simulink model "chapter2_4"  (R2022a)
settings: Solver=FixedStepAuto  StartTime=0.0  StopTime=8  FixedStep=1e-3  RelTol=1e-3
model workspace (MAT data in the model file):
  maxRandom = 1e-06
  minRandom = -1e-06
values from neighbouring files (symbols this model uses):
  A = A_set(N1-5)    [Figure2_12and2_13.m]    (also in Figure2_3.m = 10; Figure2_9and2_10and2_11.m; parameterLoadForchapter2_4.m = 0.0005; parameterLoadForchapter2_5.m = 0.0005)
  Cb = 11e3    (= 11000)    [parameterLoadForchapter2_4.m]    (also in parameterLoadForchapter2_5.m)
  Cv = 5000    [parameterLoadForchapter2_4.m]    (also in parameterLoadForchapter2_5.m)
  d = 2.6    [parameterLoadForchapter2_4.m]    (also in parameterLoadForchapter2_5.m; parameter_load3.m)
  Jb = 927.8    [parameterLoadForchapter2_4.m]    (also in parameterLoadForchapter2_5.m)
  Jv = 3044    [parameterLoadForchapter2_4.m]    (also in parameterLoadForchapter2_5.m)
  Kb = 0.267e6    (= 267000)    [parameterLoadForchapter2_4.m]    (also in parameterLoadForchapter2_5.m)
  Kv = 1.5e6    (= 1500000)    [parameterLoadForchapter2_4.m]    (also in parameterLoadForchapter2_5.m)
  L = 210/2    (= 105)    [Figure2_18_and2_19.m]    (also in Figure2_20_and2_21.m; parameterLoadForchapter2_4.m = 15.6; parameterLoadForchapter2_5.m = 210; parameter_load3.m = 210)
  Mb = 23000    [parameterLoadForchapter2_4.m]    (also in parameterLoadForchapter2_5.m)
  Mv = 4060    [parameterLoadForchapter2_4.m]    (also in parameterLoadForchapter2_5.m)
  mw = 1670    [parameterLoadForchapter2_4.m]    (also in parameterLoadForchapter2_5.m)
  Mw = 1670    [parameterLoadForchapter2_4.m]    (also in parameterLoadForchapter2_5.m)
  N1 = 0    [Mchapter2_5.m]
  N2 = N    [Figure2_10and2_11.m]    (also in Figure2_12and2_13.m = N1; Figure2_7and2_8and2_9.m = 0; Figure2_9and2_10and2_11.m = 0; Mchapter2_5.m = 0)
  r = 0.42    [parameterLoadForchapter2_4.m]    (also in parameterLoadForchapter2_5.m; parameter_load3.m)
  v = 100/3.6    (= 27.7777777778)    [Figure2_18_and2_19.m]    (also in Figure2_20_and2_21.m; parameterLoadForchapter2_4.m = 13.8888888889; parameterLoadForchapter2_5.m; parameter_load3.m)
settings Model: Creator=Spicydel  LastModifiedBy=Spicydel

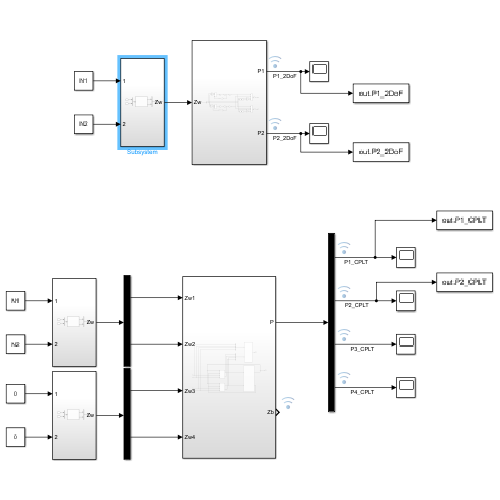
[thumbnail: Simulink's stored preview of the top-level diagram]
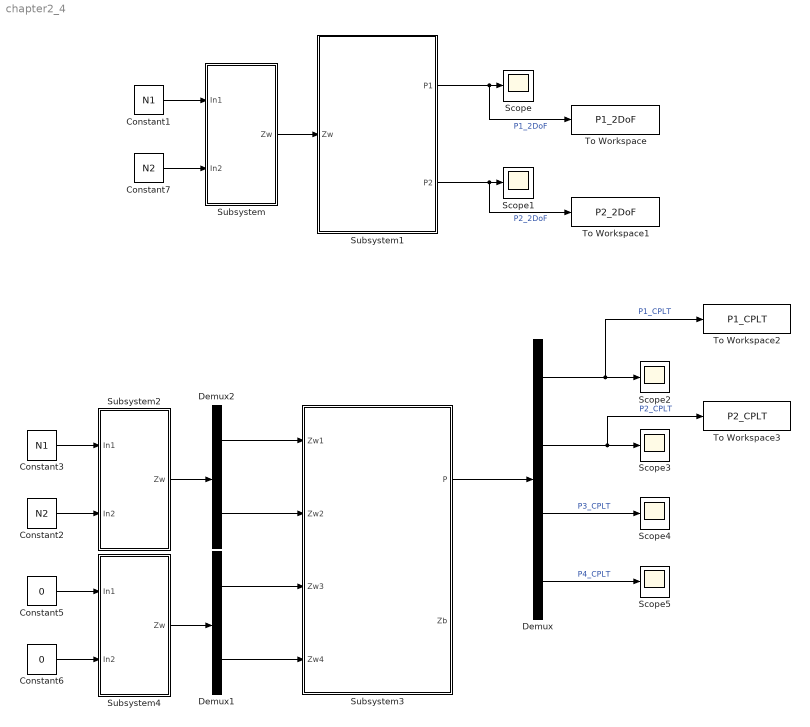
== system chapter2_4 ==
  Constant1 : Constant  Value=N1
  Constant2 : Constant  Value=N2
  Constant3 : Constant  Value=N1
  Constant5 : Constant  Value=0
  Constant6 : Constant  Value=0
  Constant7 : Constant  Value=N2
  Demux : Demux
  Demux1 : Demux  Outputs=2
  Demux2 : Demux  Outputs=2
  Scope{,1..5} (6 alike) : Scope
  Subsystem : Subsystem
  Subsystem1 : Subsystem
  Subsystem2 : Subsystem
  Subsystem3 : Subsystem
  Subsystem4 : Subsystem
  To Workspace : ToWorkspace  VariableName=P1_2DoF  SaveFormat=Timeseries  SampleTime=-1
  To Workspace1 : ToWorkspace  VariableName=P2_2DoF  SaveFormat=Timeseries  SampleTime=-1
  To Workspace2 : ToWorkspace  VariableName=P1_CPLT  SaveFormat=Timeseries  SampleTime=-1
  To Workspace3 : ToWorkspace  VariableName=P2_CPLT  SaveFormat=Timeseries  SampleTime=-1
  wires:
  Constant1/1 -> Subsystem/1(In1)
  Constant7/1 -> Subsystem/2(In2)
  Subsystem/1(Zw) -> Subsystem1/1(Zw)
  Subsystem1/1(P1) -> To Workspace/1, Scope/1  "P1_2DoF"
  Subsystem1/2(P2) -> To Workspace1/1, Scope1/1  "P2_2DoF"
  Subsystem2/1(Zw) -> Demux2/1
  Constant2/1 -> Subsystem2/2(In2)
  Constant3/1 -> Subsystem2/1(In1)
  Constant5/1 -> Subsystem4/1(In1)
  Constant6/1 -> Subsystem4/2(In2)
  Subsystem4/1(Zw) -> Demux1/1
  Demux1/1 -> Subsystem3/3(Zw3)
  Demux1/2 -> Subsystem3/4(Zw4)
  Demux2/1 -> Subsystem3/1(Zw1)
  Demux2/2 -> Subsystem3/2(Zw2)
  Subsystem3/1(P) -> Demux/1
  Demux/1 -> To Workspace2/1, Scope2/1  "P1_CPLT"
  Demux/2 -> To Workspace3/1, Scope3/1  "P2_CPLT"
  Demux/3 -> Scope4/1  "P3_CPLT"
  Demux/4 -> Scope5/1  "P4_CPLT"

== system chapter2_4/Subsystem ==
  In1 : Inport
  In2 : Inport  Port=2
  Mux1 : Mux  Inputs=2
  Mux2 : Mux  Inputs=2
  poly : Subsystem
  Zw : Outport
  wires:
  poly/1(wheel1) -> Mux2/1
  In2/1 -> Mux1/2
  poly/2(wheel2) -> Mux2/2
  Mux1/1 -> poly/1(N)
  In1/1 -> Mux1/1
  Mux2/1 -> Zw/1

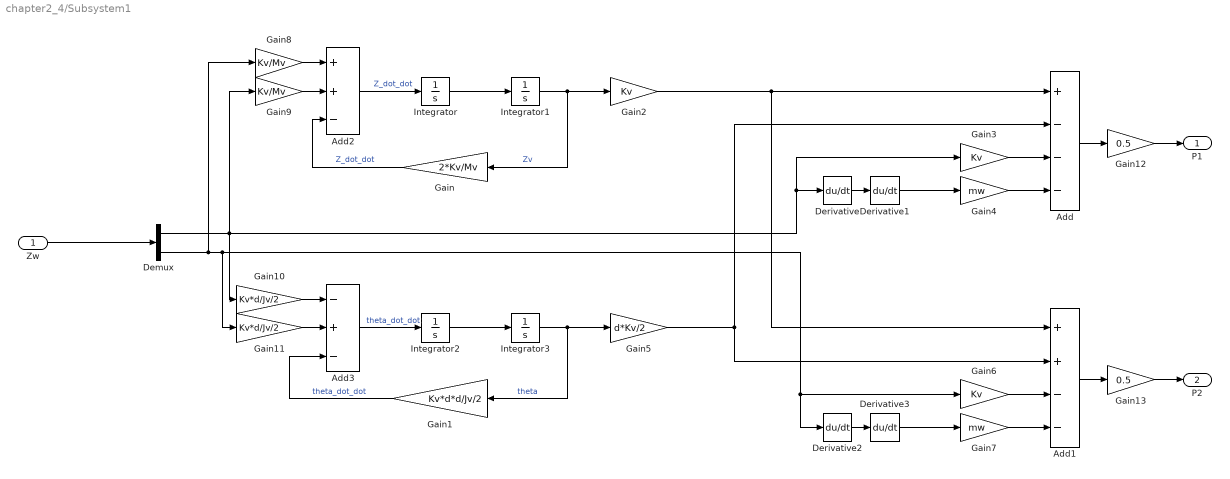
== system chapter2_4/Subsystem1 ==
  Zw : Inport
  Add : Sum  Inputs=+---
  Add1 : Sum  Inputs=++--
  Add2 : Sum  Inputs=++-
  Add3 : Sum  Inputs=-+-
  Demux : Demux  Outputs=2
  Derivative{,1..3} (4 alike) : Derivative
  Gain : Gain  Gain=2*Kv/Mv
  Gain1 : Gain  Gain=Kv*d*d/Jv/2
  Gain10 : Gain  Gain=Kv*d/Jv/2
  Gain11 : Gain  Gain=Kv*d/Jv/2
  Gain12 : Gain  Gain=0.5
  Gain13 : Gain  Gain=0.5
  Gain2 : Gain  Gain=Kv
  Gain3 : Gain  Gain=Kv
  Gain4 : Gain  Gain=mw
  Gain5 : Gain  Gain=d*Kv/2
  Gain6 : Gain  Gain=Kv
  Gain7 : Gain  Gain=mw
  Gain8 : Gain  Gain=Kv/Mv
  Gain9 : Gain  Gain=Kv/Mv
  Integrator{,1..3} (4 alike) : Integrator
  P1 : Outport
  P2 : Outport  Port=2
  wires:
  Integrator/1 -> Integrator1/1
  Integrator1/1 -> Gain2/1, Gain/1  "Zv"
  Add2/1 -> Integrator/1  "Z_dot_dot"
  Integrator2/1 -> Integrator3/1
  Integrator3/1 -> Gain5/1, Gain1/1  "theta"
  Add3/1 -> Integrator2/1  "theta_dot_dot"
  Gain2/1 -> Add1/1, Add/1
  Gain5/1 -> Add/2, Add1/2
  Add/1 -> Gain12/1
  Add1/1 -> Gain13/1
  Zw/1 -> Demux/1
  Demux/1 -> Gain10/1, Gain9/1, Derivative/1, Gain3/1
  Gain3/1 -> Add/3
  Derivative/1 -> Derivative1/1
  Derivative1/1 -> Gain4/1
  Gain4/1 -> Add/4
  Demux/2 -> Gain11/1, Gain6/1, Derivative2/1, Gain8/1
  Gain6/1 -> Add1/3
  Derivative2/1 -> Derivative3/1
  Derivative3/1 -> Gain7/1
  Gain7/1 -> Add1/4
  Gain/1 -> Add2/3  "Z_dot_dot"
  Gain8/1 -> Add2/1
  Gain9/1 -> Add2/2
  Gain1/1 -> Add3/3  "theta_dot_dot"
  Gain10/1 -> Add3/1
  Gain11/1 -> Add3/2
  Gain12/1 -> P1/1
  Gain13/1 -> P2/1

== system chapter2_4/Subsystem2 ==
  In1 : Inport
  In2 : Inport  Port=2
  Mux1 : Mux  Inputs=2
  Mux2 : Mux  Inputs=2
  poly : Subsystem
  Zw : Outport
  wires:
  Mux2/1 -> Zw/1
  In1/1 -> Mux1/1
  Mux1/1 -> poly/1(N)
  poly/2(wheel2) -> Mux2/2
  In2/1 -> Mux1/2
  poly/1(wheel1) -> Mux2/1

== system chapter2_4/Subsystem3 ==
  Zw1 : Inport
  Zw2 : Inport  Port=2
  Zw3 : Inport  Port=3
  Zw4 : Inport  Port=4
  FrontTrans : Subsystem
  Mux : Mux
  Mux1 : Mux
  RearTrans : Subsystem
  Subsystem : Subsystem
  Subsystem2 : Subsystem
  P : Outport
  Zb : Outport  Port=2
  wires:
  RearTrans/1(Zv2) -> Mux1/3, Subsystem2/2(Zv2)
  FrontTrans/1(Zv1) -> Mux1/1, Subsystem2/1(Zv1)
  Subsystem2/1(Zb) -> Zb/1, RearTrans/1(Zb), FrontTrans/1(Zb)  "Zb"
  Zw4/1 -> Mux/4, RearTrans/4(Zw4)
  Subsystem2/2(theta_b) -> FrontTrans/2(theta_b), RearTrans/2(theta_b)
  Zw3/1 -> Mux/3, RearTrans/3(Zw3)
  Zw1/1 -> Mux/1, FrontTrans/3(Zw1)
  Zw2/1 -> Mux/2, FrontTrans/4(Zw2)
  FrontTrans/2(theta_v1) -> Mux1/2
  RearTrans/2(theta_v2) -> Mux1/4
  Mux/1 -> Subsystem/1(Zw)
  Mux1/1 -> Subsystem/2(Z&theta)
  Subsystem/1(P) -> P/1

== system chapter2_4/Subsystem4 ==
  In1 : Inport
  In2 : Inport  Port=2
  Mux1 : Mux  Inputs=2
  Mux2 : Mux  Inputs=2
  poly : Subsystem
  Zw : Outport
  wires:
  poly/1(wheel1) -> Mux2/1
  In2/1 -> Mux1/2
  poly/2(wheel2) -> Mux2/2
  Mux1/1 -> poly/1(N)
  In1/1 -> Mux1/1
  Mux2/1 -> Zw/1

== system chapter2_4/Subsystem/poly ==
  N : Inport
  Clock : Clock
  Constant : Constant  Value=v
  Demux : Demux  Outputs=2
  Gain1 : Gain  Gain=1/r
  Product1 : Product
  Subsystem : Subsystem
  Subsystem1 : Subsystem
  wheel1 : Outport
  wheel2 : Outport  Port=2
  wires:
  Constant/1 -> Gain1/1
  Gain1/1 -> Product1/1
  Clock/1 -> Product1/2
  Product1/1 -> [omega]
  [omega] -> Subsystem/2(In2)
  Subsystem/1(Out1) -> wheel1/1
  [omega] -> Subsystem1/2(In2)
  Subsystem1/1(Out1) -> wheel2/1
  N/1 -> Demux/1
  Demux/1 -> Subsystem/1(In1)
  Demux/2 -> Subsystem1/1(In1)

== system chapter2_4/Subsystem2/poly ==
  N : Inport
  Clock : Clock
  Constant : Constant  Value=v
  Demux : Demux  Outputs=2
  Gain1 : Gain  Gain=1/r
  Product1 : Product
  Subsystem : Subsystem
  Subsystem1 : Subsystem
  wheel1 : Outport
  wheel2 : Outport  Port=2
  wires:
  Demux/2 -> Subsystem1/1(In1)
  Demux/1 -> Subsystem/1(In1)
  N/1 -> Demux/1
  Subsystem1/1(Out1) -> wheel2/1
  [omega] -> Subsystem1/2(In2)
  Subsystem/1(Out1) -> wheel1/1
  [omega] -> Subsystem/2(In2)
  Product1/1 -> [omega]
  Clock/1 -> Product1/2
  Gain1/1 -> Product1/1
  Constant/1 -> Gain1/1

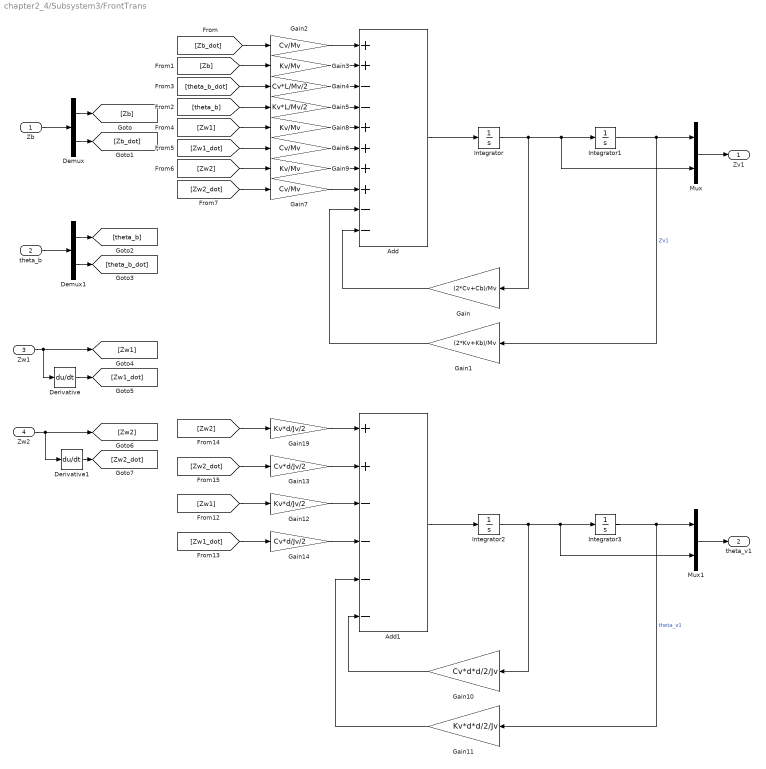
== system chapter2_4/Subsystem3/FrontTrans ==
  Zb : Inport
  theta_b : Inport  Port=2
  Zw1 : Inport  Port=3
  Zw2 : Inport  Port=4
  Add : Sum  Inputs=++--++++--
  Add1 : Sum  Inputs=++----
  Demux : Demux  Outputs=2
  Demux1 : Demux  Outputs=2
  Derivative : Derivative
  Derivative1 : Derivative
  Gain : Gain  Gain=(2*Cv+Cb)/Mv
  Gain1 : Gain  Gain=(2*Kv+Kb)/Mv
  Gain10 : Gain  Gain=Cv*d*d/2/Jv
  Gain11 : Gain  Gain=Kv*d*d/2/Jv
  Gain12 : Gain  Gain=Kv*d/Jv/2
  Gain13 : Gain  Gain=Cv*d/Jv/2
  Gain14 : Gain  Gain=Cv*d/Jv/2
  Gain19 : Gain  Gain=Kv*d/Jv/2
  Gain2 : Gain  Gain=Cv/Mv
  Gain3 : Gain  Gain=Kv/Mv
  Gain4 : Gain  Gain=Cv*L/Mv/2
  Gain5 : Gain  Gain=Kv*L/Mv/2
  Gain6 : Gain  Gain=Cv/Mv
  Gain7 : Gain  Gain=Cv/Mv
  Gain8 : Gain  Gain=Kv/Mv
  Gain9 : Gain  Gain=Kv/Mv
  Integrator{,1..3} (4 alike) : Integrator
  Mux : Mux  Inputs=2
  Mux1 : Mux  Inputs=2
  Zv1 : Outport
  theta_v1 : Outport  Port=2
  wires:
  Zb/1 -> Demux/1
  theta_b/1 -> Demux1/1
  Demux/1 -> [Zb]
  Demux/2 -> [Zb_dot]
  Demux1/1 -> [theta_b]
  Demux1/2 -> [theta_b_dot]
  Integrator/1 -> Gain/1, Mux/2, Integrator1/1
  Add/1 -> Integrator/1
  Integrator1/1 -> Gain1/1, Mux/1  "Zv1"
  Mux/1 -> Zv1/1
  Zw1/1 -> [Zw1], Derivative/1
  Gain/1 -> Add/10
  Gain1/1 -> Add/9
  [Zb_dot] -> Gain2/1
  Gain2/1 -> Add/1
  [Zb] -> Gain3/1
  Gain3/1 -> Add/2
  [theta_b_dot] -> Gain4/1
  Gain4/1 -> Add/3
  [theta_b] -> Gain5/1
  Gain5/1 -> Add/4
  [Zw2] -> Gain9/1
  [Zw2_dot] -> Gain7/1
  [Zw1_dot] -> Gain6/1
  [Zw1] -> Gain8/1
  Gain8/1 -> Add/5
  Gain6/1 -> Add/6
  Gain9/1 -> Add/7
  Gain7/1 -> Add/8
  [Zw1] -> Gain12/1
  [Zw1_dot] -> Gain14/1
  [Zw2_dot] -> Gain13/1
  [Zw2] -> Gain19/1
  Gain11/1 -> Add1/5
  Gain10/1 -> Add1/6
  Add1/1 -> Integrator2/1
  Gain19/1 -> Add1/1
  Gain12/1 -> Add1/3
  Gain13/1 -> Add1/2
  Gain14/1 -> Add1/4
  Mux1/1 -> theta_v1/1
  Integrator3/1 -> Mux1/1, Gain11/1  "theta_v1"
  Integrator2/1 -> Mux1/2, Integrator3/1, Gain10/1
  Derivative/1 -> [Zw1_dot]
  Zw2/1 -> [Zw2], Derivative1/1
  Derivative1/1 -> [Zw2_dot]

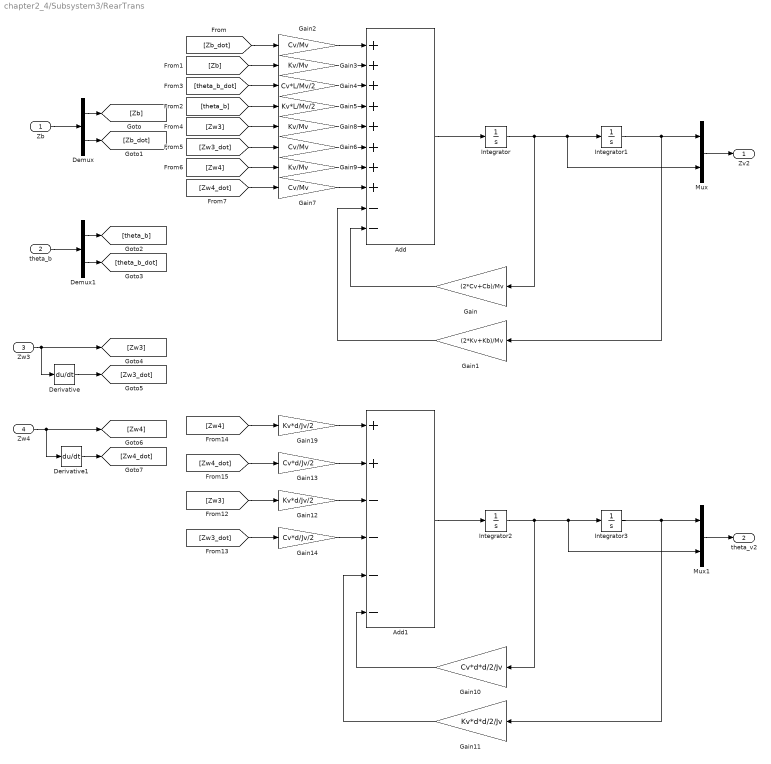
== system chapter2_4/Subsystem3/RearTrans ==
  Zb : Inport
  theta_b : Inport  Port=2
  Zw3 : Inport  Port=3
  Zw4 : Inport  Port=4
  Add : Sum  Inputs=++++++++--
  Add1 : Sum  Inputs=++----
  Demux : Demux  Outputs=2
  Demux1 : Demux  Outputs=2
  Derivative : Derivative
  Derivative1 : Derivative
  Gain : Gain  Gain=(2*Cv+Cb)/Mv
  Gain1 : Gain  Gain=(2*Kv+Kb)/Mv
  Gain10 : Gain  Gain=Cv*d*d/2/Jv
  Gain11 : Gain  Gain=Kv*d*d/2/Jv
  Gain12 : Gain  Gain=Kv*d/Jv/2
  Gain13 : Gain  Gain=Cv*d/Jv/2
  Gain14 : Gain  Gain=Cv*d/Jv/2
  Gain19 : Gain  Gain=Kv*d/Jv/2
  Gain2 : Gain  Gain=Cv/Mv
  Gain3 : Gain  Gain=Kv/Mv
  Gain4 : Gain  Gain=Cv*L/Mv/2
  Gain5 : Gain  Gain=Kv*L/Mv/2
  Gain6 : Gain  Gain=Cv/Mv
  Gain7 : Gain  Gain=Cv/Mv
  Gain8 : Gain  Gain=Kv/Mv
  Gain9 : Gain  Gain=Kv/Mv
  Integrator{,1..3} (4 alike) : Integrator
  Mux : Mux  Inputs=2
  Mux1 : Mux  Inputs=2
  Zv2 : Outport
  theta_v2 : Outport  Port=2
  wires:
  Gain14/1 -> Add1/4
  Gain13/1 -> Add1/2
  Gain12/1 -> Add1/3
  Gain19/1 -> Add1/1
  Add1/1 -> Integrator2/1
  Gain10/1 -> Add1/6
  Gain11/1 -> Add1/5
  [Zw4] -> Gain19/1
  [Zw4_dot] -> Gain13/1
  [Zw3_dot] -> Gain14/1
  [Zw3] -> Gain12/1
  Gain7/1 -> Add/8
  Gain9/1 -> Add/7
  Gain6/1 -> Add/6
  Gain8/1 -> Add/5
  [Zw3] -> Gain8/1
  [Zw3_dot] -> Gain6/1
  [Zw4_dot] -> Gain7/1
  [Zw4] -> Gain9/1
  Gain5/1 -> Add/4
  [theta_b] -> Gain5/1
  Gain4/1 -> Add/3
  [theta_b_dot] -> Gain4/1
  Gain3/1 -> Add/2
  [Zb] -> Gain3/1
  Gain2/1 -> Add/1
  [Zb_dot] -> Gain2/1
  Gain1/1 -> Add/9
  Gain/1 -> Add/10
  Zw4/1 -> Derivative1/1, [Zw4]
  Derivative1/1 -> [Zw4_dot]
  Zw3/1 -> Derivative/1, [Zw3]
  Mux/1 -> Zv2/1
  Integrator1/1 -> Mux/1, Gain1/1
  Add/1 -> Integrator/1
  Integrator/1 -> Integrator1/1, Mux/2, Gain/1
  Demux1/2 -> [theta_b_dot]
  Demux1/1 -> [theta_b]
  Demux/2 -> [Zb_dot]
  Demux/1 -> [Zb]
  theta_b/1 -> Demux1/1
  Zb/1 -> Demux/1
  Integrator2/1 -> Gain10/1, Mux1/2, Integrator3/1
  Integrator3/1 -> Mux1/1, Gain11/1
  Mux1/1 -> theta_v2/1
  Derivative/1 -> [Zw3_dot]

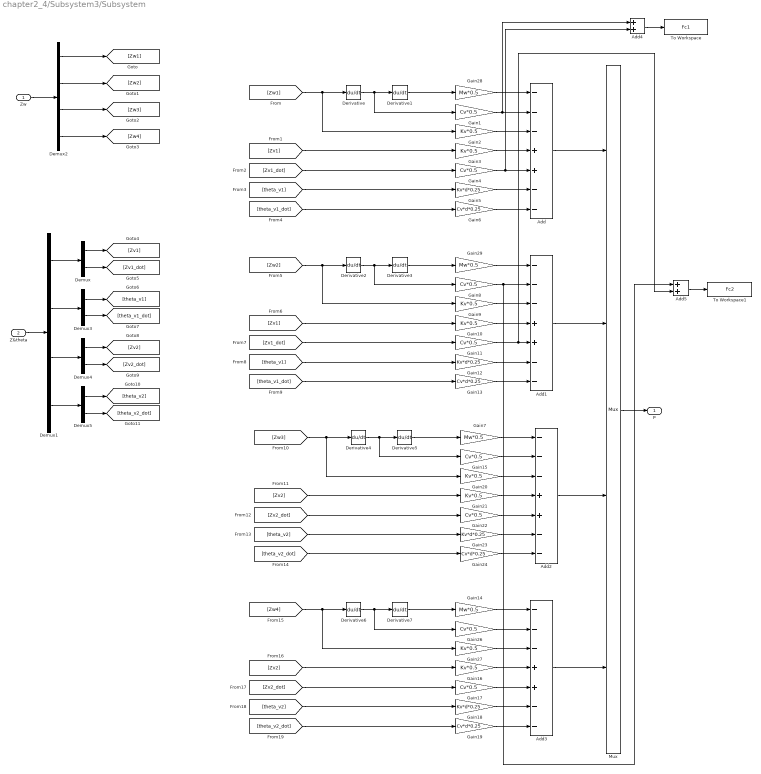
== system chapter2_4/Subsystem3/Subsystem ==
  Zw : Inport
  Z&theta : Inport  Port=2
  Add{,1..3} (4 alike) : Sum  Inputs=---++--
  Add4 : Sum
  Add5 : Sum
  Demux{,3..5} (4 alike) : Demux  Outputs=2
  Demux1 : Demux
  Demux2 : Demux
  Derivative{,1..7} (8 alike) : Derivative
  Gain{1,4,8,11,15,17,22,26} (8 alike) : Gain  Gain=Cv*0.5
  Gain{2..3,9..10,16,20..21,27} (8 alike) : Gain  Gain=Kv*0.5
  Gain{5,12,18,23} (4 alike) : Gain  Gain=Kv*d*0.25
  Gain{6,13,19,24} (4 alike) : Gain  Gain=Cv*d*0.25
  Gain{7,14,28..29} (4 alike) : Gain  Gain=Mw*0.5
  Mux : Mux
  To Workspace : ToWorkspace  VariableName=Fc1  SaveFormat=Timeseries  SampleTime=-1
  To Workspace1 : ToWorkspace  VariableName=Fc2  SaveFormat=Timeseries  SampleTime=-1
  P : Outport
  wires:
  Zw/1 -> Demux2/1
  Z&theta/1 -> Demux1/1
  Demux2/1 -> [Zw1]
  Demux2/2 -> [Zw2]
  Demux2/3 -> [Zw3]
  Demux2/4 -> [Zw4]
  Demux1/1 -> Demux/1
  Demux1/2 -> Demux3/1
  Demux1/3 -> Demux4/1
  Demux1/4 -> Demux5/1
  Demux/1 -> [Zv1]
  Demux/2 -> [Zv1_dot]
  Demux3/1 -> [theta_v1]
  Demux3/2 -> [theta_v1_dot]
  Demux4/2 -> [Zv2_dot]
  Demux4/1 -> [Zv2]
  Demux5/2 -> [theta_v2_dot]
  Demux5/1 -> [theta_v2]
  [Zw1] -> Gain2/1, Derivative/1
  Derivative/1 -> Gain1/1, Derivative1/1
  Derivative1/1 -> Gain28/1
  Gain28/1 -> Add/1
  Gain1/1 -> Add4/1, Add/2
  Gain2/1 -> Add/3
  Gain3/1 -> Add/4
  [Zv1] -> Gain3/1
  Gain4/1 -> Add4/2, Add/5
  [Zv1_dot] -> Gain4/1
  Gain5/1 -> Add/6
  Gain6/1 -> Add/7
  [theta_v1] -> Gain5/1
  [theta_v1_dot] -> Gain6/1
  Add/1 -> Mux/1
  Add1/1 -> Mux/2
  [theta_v1_dot] -> Gain13/1
  [theta_v1] -> Gain12/1
  Gain13/1 -> Add1/7
  Gain12/1 -> Add1/6
  [Zv1_dot] -> Gain11/1
  Gain11/1 -> Add5/2, Add1/5
  [Zv1] -> Gain10/1
  Gain10/1 -> Add1/4
  Gain9/1 -> Add1/3
  Gain8/1 -> Add5/1, Add1/2
  Gain29/1 -> Add1/1
  Derivative3/1 -> Gain29/1
  Derivative2/1 -> Derivative3/1, Gain8/1
  [Zw2] -> Gain9/1, Derivative2/1
  [Zw4] -> Gain27/1, Derivative6/1
  Derivative6/1 -> Gain26/1, Derivative7/1
  Derivative7/1 -> Gain14/1
  Gain14/1 -> Add3/1
  Gain26/1 -> Add3/2
  Gain27/1 -> Add3/3
  Gain16/1 -> Add3/4
  [Zv2] -> Gain16/1
  Gain17/1 -> Add3/5
  [Zv2_dot] -> Gain17/1
  Gain18/1 -> Add3/6
  Gain19/1 -> Add3/7
  [theta_v2] -> Gain18/1
  [theta_v2_dot] -> Gain19/1
  Add3/1 -> Mux/4
  Add2/1 -> Mux/3
  [theta_v2_dot] -> Gain24/1
  [theta_v2] -> Gain23/1
  Gain24/1 -> Add2/7
  Gain23/1 -> Add2/6
  [Zv2_dot] -> Gain22/1
  Gain22/1 -> Add2/5
  [Zv2] -> Gain21/1
  Gain21/1 -> Add2/4
  Gain20/1 -> Add2/3
  Gain15/1 -> Add2/2
  Gain7/1 -> Add2/1
  Derivative5/1 -> Gain7/1
  Derivative4/1 -> Derivative5/1, Gain15/1
  [Zw3] -> Gain20/1, Derivative4/1
  Mux/1 -> P/1
  Add4/1 -> To Workspace/1
  Add5/1 -> To Workspace1/1

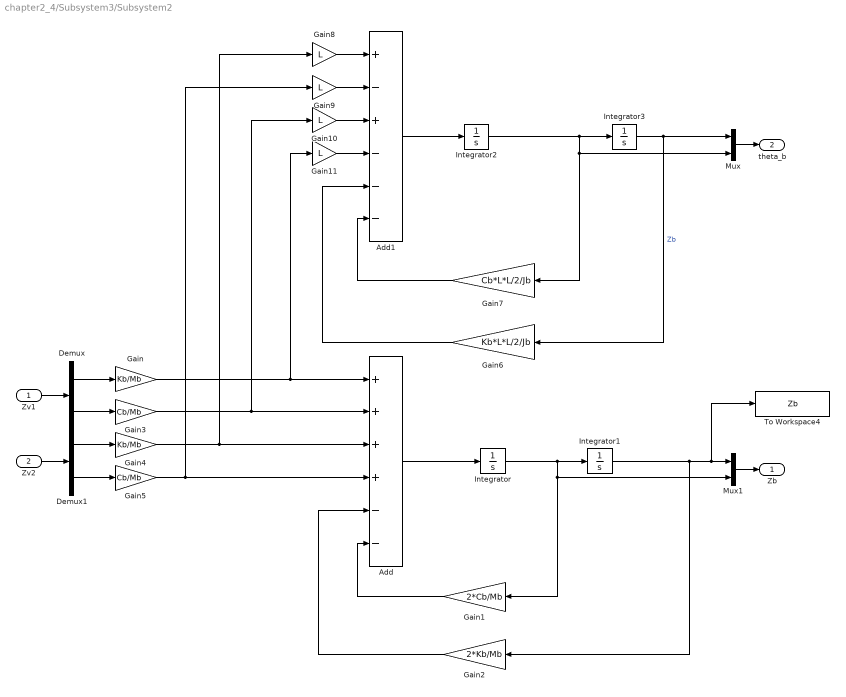
== system chapter2_4/Subsystem3/Subsystem2 ==
  Zv1 : Inport
  Zv2 : Inport  Port=2
  Add : Sum  Inputs=++++--
  Add1 : Sum  Inputs=+-+---
  Demux : Demux  Outputs=2
  Demux1 : Demux  Outputs=2
  Gain : Gain  Gain=Kb/Mb
  Gain1 : Gain  Gain=2*Cb/Mb
  Gain{8..11} (4 alike) : Gain  Gain=L
  Gain2 : Gain  Gain=2*Kb/Mb
  Gain3 : Gain  Gain=Cb/Mb
  Gain4 : Gain  Gain=Kb/Mb
  Gain5 : Gain  Gain=Cb/Mb
  Gain6 : Gain  Gain=Kb*L*L/2/Jb
  Gain7 : Gain  Gain=Cb*L*L/2/Jb
  Integrator{,1..3} (4 alike) : Integrator
  Mux : Mux  Inputs=2
  Mux1 : Mux  Inputs=2
  To Workspace4 : ToWorkspace  VariableName=Zb  SaveFormat=Timeseries  SampleTime=-1
  Zb : Outport
  theta_b : Outport  Port=2
  wires:
  Gain1/1 -> Add/6
  Add/1 -> Integrator/1
  Gain2/1 -> Add/5
  Integrator/1 -> Mux1/2, Gain1/1, Integrator1/1
  Integrator1/1 -> To Workspace4/1, Mux1/1, Gain2/1
  Gain/1 -> Gain11/1, Add/1
  Gain4/1 -> Gain8/1, Add/3
  Gain5/1 -> Gain9/1, Add/4
  Integrator2/1 -> Mux/2, Gain7/1, Integrator3/1
  Integrator3/1 -> Mux/1, Gain6/1  "Zb"
  Add1/1 -> Integrator2/1
  Gain7/1 -> Add1/6
  Gain6/1 -> Add1/5
  Gain3/1 -> Gain10/1, Add/2
  Gain8/1 -> Add1/1
  Gain9/1 -> Add1/2
  Gain10/1 -> Add1/3
  Gain11/1 -> Add1/4
  Mux/1 -> theta_b/1
  Mux1/1 -> Zb/1
  Zv1/1 -> Demux/1
  Demux/1 -> Gain/1
  Demux/2 -> Gain3/1
  Zv2/1 -> Demux1/1
  Demux1/1 -> Gain4/1
  Demux1/2 -> Gain5/1

== system chapter2_4/Subsystem4/poly ==
  N : Inport
  Clock : Clock
  Constant : Constant  Value=v
  Demux : Demux  Outputs=2
  Gain1 : Gain  Gain=1/r
  Product1 : Product
  Subsystem : Subsystem
  Subsystem1 : Subsystem
  wheel1 : Outport
  wheel2 : Outport  Port=2
  wires:
  Constant/1 -> Gain1/1
  Gain1/1 -> Product1/1
  Clock/1 -> Product1/2
  Product1/1 -> [omega]
  [omega] -> Subsystem/2(In2)
  Subsystem/1(Out1) -> wheel1/1
  [omega] -> Subsystem1/2(In2)
  Subsystem1/1(Out1) -> wheel2/1
  N/1 -> Demux/1
  Demux/1 -> Subsystem/1(In1)
  Demux/2 -> Subsystem1/1(In1)

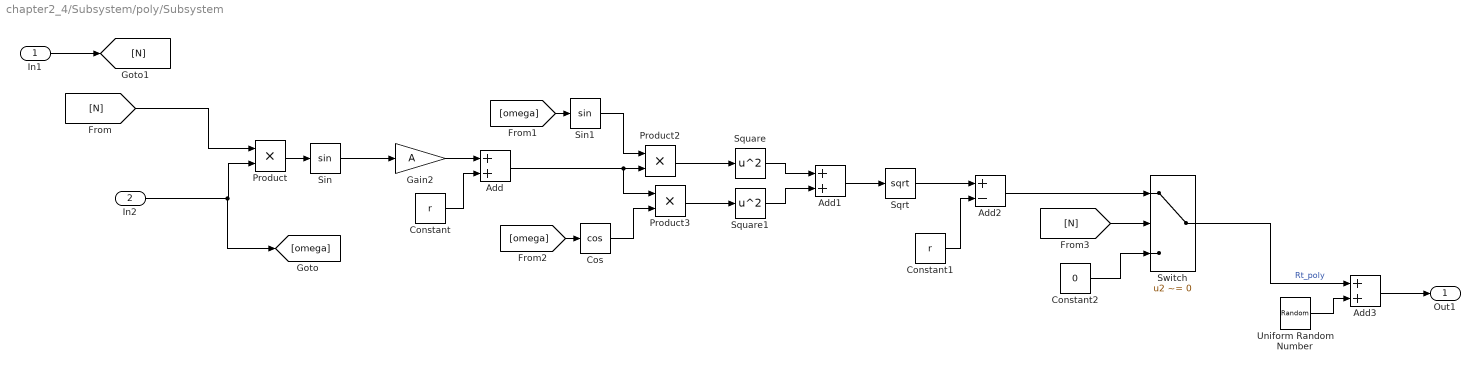
== system chapter2_4/Subsystem/poly/Subsystem ==
  In1 : Inport
  In2 : Inport  Port=2
  Add : Sum
  Add1 : Sum
  Add2 : Sum  Inputs=+-
  Add3 : Sum
  Constant : Constant  Value=r
  Constant1 : Constant  Value=r
  Constant2 : Constant  Value=0
  Cos : Trigonometry  Operator=cos
  Gain2 : Gain  Gain=A
  Product : Product
  Product2 : Product
  Product3 : Product
  Sin : Trigonometry
  Sin1 : Trigonometry
  Sqrt : Sqrt
  Square : Math  Operator=square
  Square1 : Math  Operator=square
  Switch : Switch  Criteria=u2 ~= 0  SaturateOnIntegerOverflow=off  InputSameDT=off
  Uniform Random Number : UniformRandomNumber  Minimum=minRandom  Maximum=maxRandom  SampleTime=1e-3
  Out1 : Outport
  wires:
  Cos/1 -> Product3/2
  Product/1 -> Sin/1
  Sin/1 -> Gain2/1
  Gain2/1 -> Add/1
  Add/1 -> Product3/1, Product2/2
  Constant/1 -> Add/2
  [omega] -> Sin1/1
  Sin1/1 -> Product2/1
  [omega] -> Cos/1
  Product2/1 -> Square/1
  Constant1/1 -> Add2/2
  Sqrt/1 -> Add2/1
  Square1/1 -> Add1/2
  Product3/1 -> Square1/1
  Square/1 -> Add1/1
  Add1/1 -> Sqrt/1
  In2/1 -> [omega], Product/2
  [N] -> Product/1
  In1/1 -> [N]
  [N] -> Switch/2
  Switch/1 -> Add3/1  "Rt_poly"
  Add2/1 -> Switch/1
  Constant2/1 -> Switch/3
  Uniform Random Number/1 -> Add3/2
  Add3/1 -> Out1/1

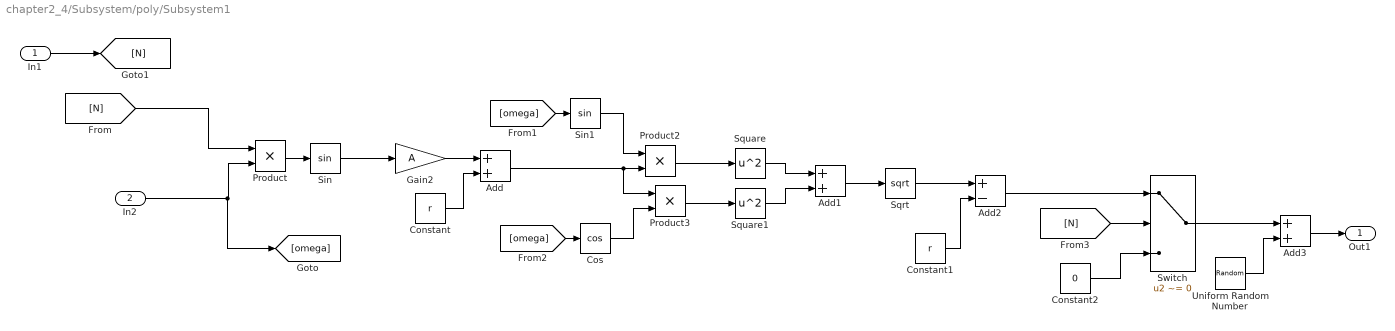
== system chapter2_4/Subsystem/poly/Subsystem1 ==
  In1 : Inport
  In2 : Inport  Port=2
  Add : Sum
  Add1 : Sum
  Add2 : Sum  Inputs=+-
  Add3 : Sum
  Constant : Constant  Value=r
  Constant1 : Constant  Value=r
  Constant2 : Constant  Value=0
  Cos : Trigonometry  Operator=cos
  Gain2 : Gain  Gain=A
  Product : Product
  Product2 : Product
  Product3 : Product
  Sin : Trigonometry
  Sin1 : Trigonometry
  Sqrt : Sqrt
  Square : Math  Operator=square
  Square1 : Math  Operator=square
  Switch : Switch  Criteria=u2 ~= 0  SaturateOnIntegerOverflow=off  InputSameDT=off
  Uniform Random Number : UniformRandomNumber  Minimum=minRandom  Maximum=maxRandom  Seed=3  SampleTime=1e-3
  Out1 : Outport
  wires:
  Constant2/1 -> Switch/3
  Add2/1 -> Switch/1
  Switch/1 -> Add3/1
  [N] -> Switch/2
  In1/1 -> [N]
  [N] -> Product/1
  In2/1 -> Product/2, [omega]
  Add1/1 -> Sqrt/1
  Square/1 -> Add1/1
  Product3/1 -> Square1/1
  Square1/1 -> Add1/2
  Sqrt/1 -> Add2/1
  Constant1/1 -> Add2/2
  Product2/1 -> Square/1
  [omega] -> Cos/1
  Sin1/1 -> Product2/1
  [omega] -> Sin1/1
  Constant/1 -> Add/2
  Add/1 -> Product2/2, Product3/1
  Gain2/1 -> Add/1
  Sin/1 -> Gain2/1
  Product/1 -> Sin/1
  Cos/1 -> Product3/2
  Uniform Random Number/1 -> Add3/2
  Add3/1 -> Out1/1

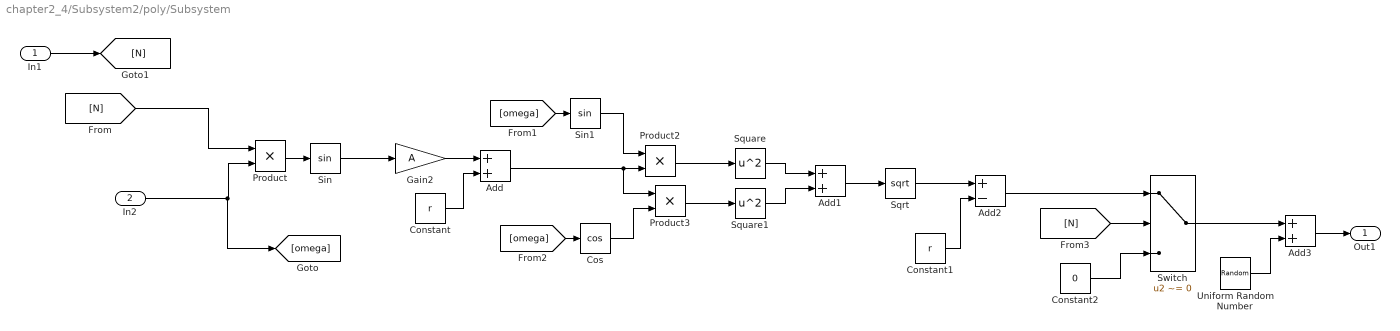
== system chapter2_4/Subsystem2/poly/Subsystem ==
  In1 : Inport
  In2 : Inport  Port=2
  Add : Sum
  Add1 : Sum
  Add2 : Sum  Inputs=+-
  Add3 : Sum
  Constant : Constant  Value=r
  Constant1 : Constant  Value=r
  Constant2 : Constant  Value=0
  Cos : Trigonometry  Operator=cos
  Gain2 : Gain  Gain=A
  Product : Product
  Product2 : Product
  Product3 : Product
  Sin : Trigonometry
  Sin1 : Trigonometry
  Sqrt : Sqrt
  Square : Math  Operator=square
  Square1 : Math  Operator=square
  Switch : Switch  Criteria=u2 ~= 0  SaturateOnIntegerOverflow=off  InputSameDT=off
  Uniform Random Number : UniformRandomNumber  Minimum=minRandom  Maximum=maxRandom  Seed=4  SampleTime=1e-3
  Out1 : Outport
  wires:
  Constant2/1 -> Switch/3
  Add2/1 -> Switch/1
  Switch/1 -> Add3/1
  [N] -> Switch/2
  In1/1 -> [N]
  [N] -> Product/1
  In2/1 -> Product/2, [omega]
  Add1/1 -> Sqrt/1
  Square/1 -> Add1/1
  Product3/1 -> Square1/1
  Square1/1 -> Add1/2
  Sqrt/1 -> Add2/1
  Constant1/1 -> Add2/2
  Product2/1 -> Square/1
  [omega] -> Cos/1
  Sin1/1 -> Product2/1
  [omega] -> Sin1/1
  Constant/1 -> Add/2
  Add/1 -> Product2/2, Product3/1
  Gain2/1 -> Add/1
  Sin/1 -> Gain2/1
  Product/1 -> Sin/1
  Cos/1 -> Product3/2
  Uniform Random Number/1 -> Add3/2
  Add3/1 -> Out1/1

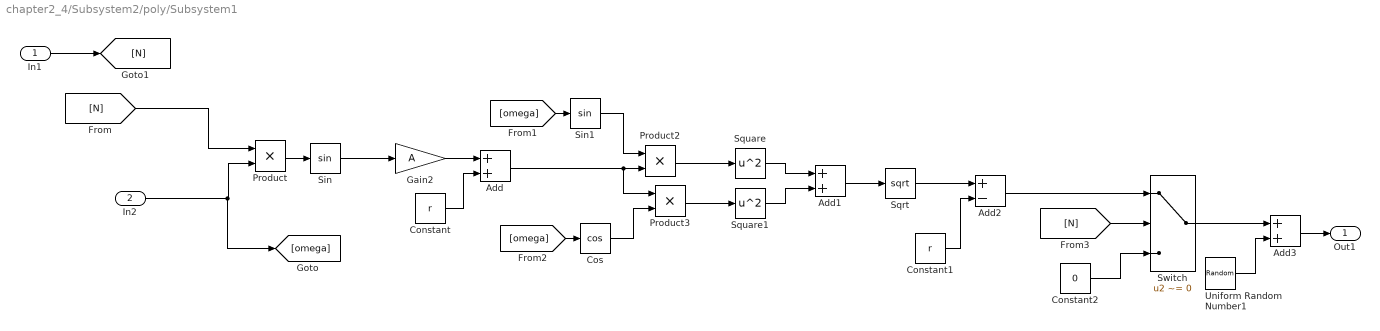
== system chapter2_4/Subsystem2/poly/Subsystem1 ==
  In1 : Inport
  In2 : Inport  Port=2
  Add : Sum
  Add1 : Sum
  Add2 : Sum  Inputs=+-
  Add3 : Sum
  Constant : Constant  Value=r
  Constant1 : Constant  Value=r
  Constant2 : Constant  Value=0
  Cos : Trigonometry  Operator=cos
  Gain2 : Gain  Gain=A
  Product : Product
  Product2 : Product
  Product3 : Product
  Sin : Trigonometry
  Sin1 : Trigonometry
  Sqrt : Sqrt
  Square : Math  Operator=square
  Square1 : Math  Operator=square
  Switch : Switch  Criteria=u2 ~= 0  SaturateOnIntegerOverflow=off  InputSameDT=off
  Uniform Random Number1 : UniformRandomNumber  Minimum=minRandom  Maximum=maxRandom  Seed=3  SampleTime=1e-3
  Out1 : Outport
  wires:
  Cos/1 -> Product3/2
  Product/1 -> Sin/1
  Sin/1 -> Gain2/1
  Gain2/1 -> Add/1
  Add/1 -> Product3/1, Product2/2
  Constant/1 -> Add/2
  [omega] -> Sin1/1
  Sin1/1 -> Product2/1
  [omega] -> Cos/1
  Product2/1 -> Square/1
  Constant1/1 -> Add2/2
  Sqrt/1 -> Add2/1
  Square1/1 -> Add1/2
  Product3/1 -> Square1/1
  Square/1 -> Add1/1
  Add1/1 -> Sqrt/1
  In2/1 -> [omega], Product/2
  [N] -> Product/1
  In1/1 -> [N]
  [N] -> Switch/2
  Switch/1 -> Add3/1
  Add2/1 -> Switch/1
  Constant2/1 -> Switch/3
  Uniform Random Number1/1 -> Add3/2
  Add3/1 -> Out1/1

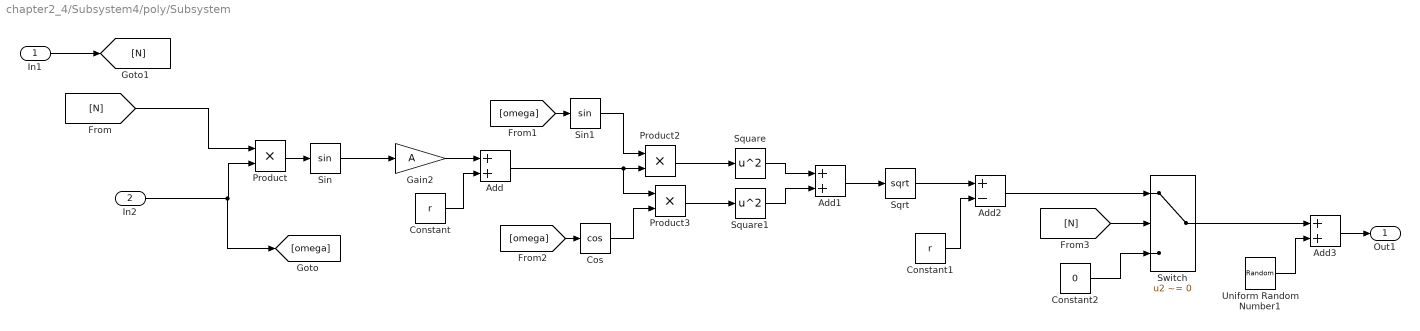
== system chapter2_4/Subsystem4/poly/Subsystem ==
  In1 : Inport
  In2 : Inport  Port=2
  Add : Sum
  Add1 : Sum
  Add2 : Sum  Inputs=+-
  Add3 : Sum
  Constant : Constant  Value=r
  Constant1 : Constant  Value=r
  Constant2 : Constant  Value=0
  Cos : Trigonometry  Operator=cos
  Gain2 : Gain  Gain=A
  Product : Product
  Product2 : Product
  Product3 : Product
  Sin : Trigonometry
  Sin1 : Trigonometry
  Sqrt : Sqrt
  Square : Math  Operator=square
  Square1 : Math  Operator=square
  Switch : Switch  Criteria=u2 ~= 0  SaturateOnIntegerOverflow=off  InputSameDT=off
  Uniform Random Number1 : UniformRandomNumber  Minimum=minRandom  Maximum=maxRandom  Seed=2  SampleTime=1e-3
  Out1 : Outport
  wires:
  Cos/1 -> Product3/2
  Product/1 -> Sin/1
  Sin/1 -> Gain2/1
  Gain2/1 -> Add/1
  Add/1 -> Product3/1, Product2/2
  Constant/1 -> Add/2
  [omega] -> Sin1/1
  Sin1/1 -> Product2/1
  [omega] -> Cos/1
  Product2/1 -> Square/1
  Constant1/1 -> Add2/2
  Sqrt/1 -> Add2/1
  Square1/1 -> Add1/2
  Product3/1 -> Square1/1
  Square/1 -> Add1/1
  Add1/1 -> Sqrt/1
  In2/1 -> [omega], Product/2
  [N] -> Product/1
  In1/1 -> [N]
  [N] -> Switch/2
  Switch/1 -> Add3/1
  Add2/1 -> Switch/1
  Constant2/1 -> Switch/3
  Uniform Random Number1/1 -> Add3/2
  Add3/1 -> Out1/1

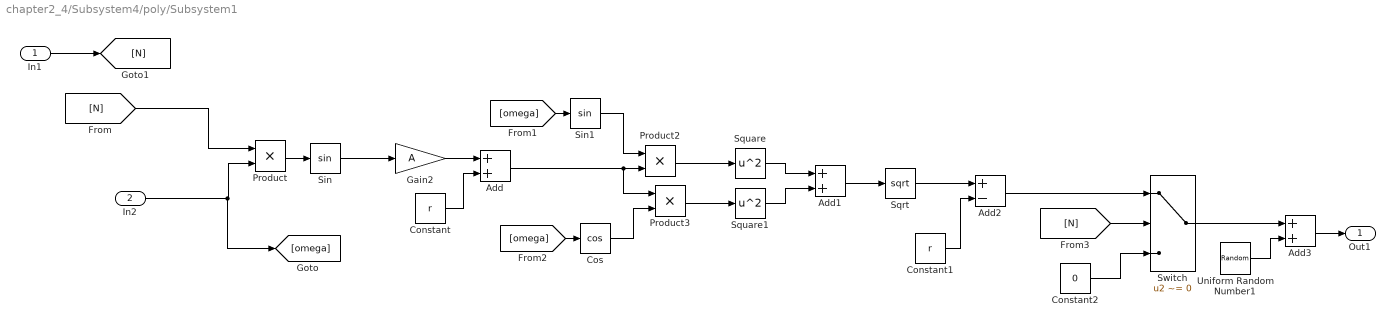
== system chapter2_4/Subsystem4/poly/Subsystem1 ==
  In1 : Inport
  In2 : Inport  Port=2
  Add : Sum
  Add1 : Sum
  Add2 : Sum  Inputs=+-
  Add3 : Sum
  Constant : Constant  Value=r
  Constant1 : Constant  Value=r
  Constant2 : Constant  Value=0
  Cos : Trigonometry  Operator=cos
  Gain2 : Gain  Gain=A
  Product : Product
  Product2 : Product
  Product3 : Product
  Sin : Trigonometry
  Sin1 : Trigonometry
  Sqrt : Sqrt
  Square : Math  Operator=square
  Square1 : Math  Operator=square
  Switch : Switch  Criteria=u2 ~= 0  SaturateOnIntegerOverflow=off  InputSameDT=off
  Uniform Random Number1 : UniformRandomNumber  Minimum=minRandom  Maximum=maxRandom  Seed=1  SampleTime=1e-3
  Out1 : Outport
  wires:
  Constant2/1 -> Switch/3
  Add2/1 -> Switch/1
  Switch/1 -> Add3/1
  [N] -> Switch/2
  In1/1 -> [N]
  [N] -> Product/1
  In2/1 -> Product/2, [omega]
  Add1/1 -> Sqrt/1
  Square/1 -> Add1/1
  Product3/1 -> Square1/1
  Square1/1 -> Add1/2
  Sqrt/1 -> Add2/1
  Constant1/1 -> Add2/2
  Product2/1 -> Square/1
  [omega] -> Cos/1
  Sin1/1 -> Product2/1
  [omega] -> Sin1/1
  Constant/1 -> Add/2
  Add/1 -> Product2/2, Product3/1
  Gain2/1 -> Add/1
  Sin/1 -> Gain2/1
  Product/1 -> Sin/1
  Cos/1 -> Product3/2
  Uniform Random Number1/1 -> Add3/2
  Add3/1 -> Out1/1
